simulink model "PID_DC_motor_control_linear"  (R2017a)
settings: Solver=ode45  StartTime=0.0  StopTime=50  RelTol=1e-5  EnableMultiTasking=on
libraries: simulink x1
settings Model: Creator=The MathWorks, Inc.  LastModifiedBy=hemma
settings DataIOCC: LimitDataPoints=on  SaveFormat=Array
settings OptimizationCC: ExpressionDepthLimit=2147483647  LifeSpan=inf
settings DebuggingCC: UnderspecifiedInitializationDetection=Classic  MergeDetectMultiDrivingBlocksExec=none  FcnCallInpInsideContextMsg=warning  AllowSymbolicDim=off  StateNameClashWarn=warning  SFUnexpectedBacktrackingDiag=warning  SFNoUnconditionalDefaultTransitionDiag=warning  SFExecutionAtInitializationDiag=none
settings HardwareCC: ProdBitPerPointer=32  ProdBitPerSizeT=32  ProdBitPerPtrDiffT=32  ProdLargestAtomicFloat=None  ProdIntDivRoundTo=Undefined  ProdEndianess=Unspecified  ProdWordSize=32  ProdHWDeviceType=32-bit Generic
settings ModelReferenceCC: PropagateSignalLabelsOutOfModel=off
settings GRTTargetCC: TargetLangStandard=C89/C90 (ANSI)  GeneratePreprocessorConditionals=Disable all  CombineOutputUpdateFcns=off  GRTInterface=on
settings ConfigComp: CovMetricSettings=dw  CovHtmlReporting=on  CovSaveCumulativeToWorkspaceVar=on  CovSaveSingleToWorkspaceVar=on  CovExternalEMLEnable=off  CovSFcnEnable=off

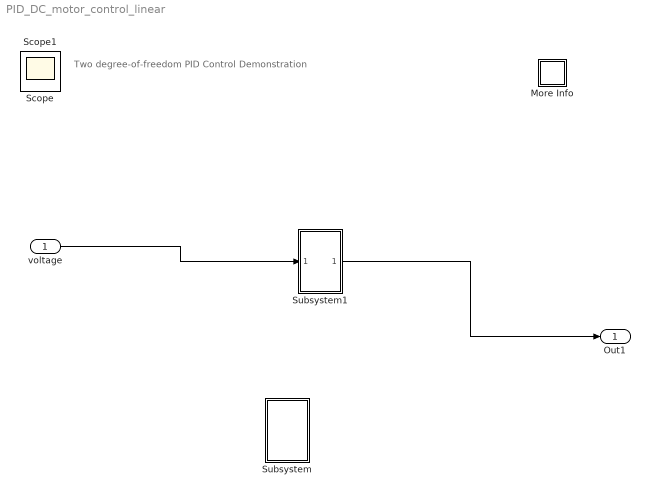
== system PID_DC_motor_control_linear ==
  note: Two degree-of-freedom PID Control Demonstration
  "voltage " : Inport
  More Info : Subsystem
      settings: OpenFcn=showdemo('sldemo_pid2dof')
      mask Display: disp('?')
  Subsystem : Subsystem
  Subsystem1 : Subsystem
  Out1 : Outport
  Scope : Scope
  Scope1 : Scope
  wires:
  "voltage "/1 -> Subsystem1/1("voltage ")
  Subsystem1/1(Out1) -> Out1/1

== system PID_DC_motor_control_linear/More Info ==

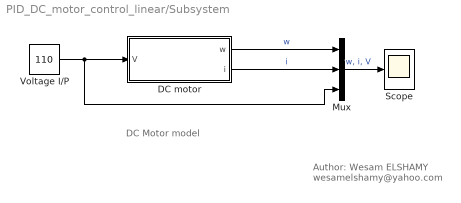
== system PID_DC_motor_control_linear/Subsystem ==
  note: Author: Wesam ELSHAMY
      | wesamelshamy@yahoo.com
  note: DC Motor model
  DC motor : Subsystem  mask(DC Motor){L=0.1, Kphi=0.3, J=0.1, b=0.01, R=2}
      mask help:
      | Takes the DC voltage as input, and outputs angular velocity (w) and current (i)
      | L => windings inductance		Kphi => emf constant
      | J => loads moment of inertial		b => viscous friction
      | R => windings resistance
      mask Display:
      | port_label('input', 1, 'V')
      | port_label('output', 2, 'i')
      | port_label('output', 1, 'w')
      | disp('DC Motor')
  Mux : Mux  Inputs=3
  Scope : Scope
  Voltage I/P : Constant  Value=110
  wires:
  DC motor/2(i) -> Mux/2  "i"
  Mux/1 -> Scope/1  "w, i, V"
  DC motor/1(w) -> Mux/1  "w"
  Voltage I/P/1 -> Mux/3, DC motor/1(V)

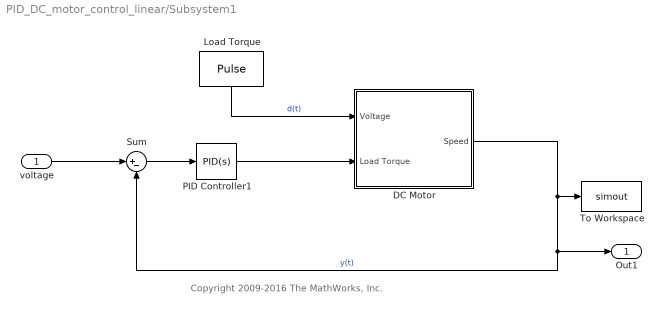
== system PID_DC_motor_control_linear/Subsystem1 ==
  note: Copyright 2009-2016 The MathWorks, Inc.
  "voltage " : Inport
  DC Motor : Subsystem  mask(DC Motor){R=2, L=0.5, Km=0.1, Kf=0.2, J=0.02, Kb=0.1}
      mask prompts: R "R (Ohms)"; L "L (Henrys)"; Km "Km (Torque Constant)"; Kf "Kf (Nms)"; J "J (kg.m^2/s^2)"; Kb "Kb (Back emf Constant)"
      mask help: An ideal model of a DC Motor
      mask Help: This is <b>more elaborate<b> help.
      mask Display: image(fullfile(matlabroot,'toolbox','simulink','simdemos','industrial','images','maskIconDCMotor.png'))
  Load Torque : DiscretePulseGenerator  PulseType=Time based  Amplitude=-20  Period=100  PulseWidth=50
  PID Controller1 : simulink/Continuous/PID Controller  Controller=PID  TimeDomain=Continuous-time  SampleTime=-1  IntegratorMethod=Forward Euler  FilterMethod=Forward Euler  Form=Parallel  UseFilter=on  ControllerParametersSource=internal  P=1.25  I=0  D=0.1  N=0  InitialConditionSource=internal  InitialConditionForIntegrator=0  InitialConditionForFilter=0  ExternalReset=none  LimitOutput=off  UpperSaturationLimit=inf  LowerSaturationLimit=-inf  LinearizeAsGain=on  AntiWindupMode=none  Kb=1  TrackingMode=off  Kt=1  PParamMin=[]  PParamMax=[]  IParamMin=[]  IParamMax=[]  DParamMin=[]  DParamMax=[]  NParamMin=[]  NParamMax=[]  KbParamMin=[]  KbParamMax=[]  KtParamMin=[]  KtParamMax=[]  POutMin=[]  POutMax=[]  IOutMin=[]  IOutMax=[]  DOutMin=[]  DOutMax=[]  NOutMin=[]  NOutMax=[]  KbOutMin=[]  KbOutMax=[]  KtOutMin=[]  KtOutMax=[]  IntegratorOutMin=[]  IntegratorOutMax=[]  FilterOutMin=[]  FilterOutMax=[]  SumOutMin=[]  SumOutMax=[]  SumI1OutMin=[]  SumI1OutMax=[]  SumI2OutMin=[]  SumI2OutMax=[]  SumI3OutMin=[]  SumI3OutMax=[]  SumDOutMin=[]  SumDOutMax=[]  SaturationOutMin=[]  SaturationOutMax=[]  IntegratorContinuousStateAttributes=''  IntegratorStateMustResolveToSignalObject=off  IntegratorRTWStateStorageClass=Auto  FilterContinuousStateAttributes=''  FilterStateMustResolveToSignalObject=off  FilterRTWStateStorageClass=Auto  DifferentiatorICPrevScaledInput=0  DifferentiatorOutMin=[]  DifferentiatorOutMax=[]  InitialConditionSetting=State (most efficient)
  Sum : Sum  Inputs=|+-
  To Workspace : ToWorkspace  VariableName=simout  SaveFormat=Structure With Time  SampleTime=-1
  Out1 : Outport
  wires:
  Load Torque/1 -> DC Motor/1(Voltage)  "d(t)"
  "voltage "/1 -> Sum/1
  PID Controller1/1 -> DC Motor/2(Load Torque)
  DC Motor/1(Speed) -> To Workspace/1, Out1/1, Sum/2  "y(t)"
  Sum/1 -> PID Controller1/1

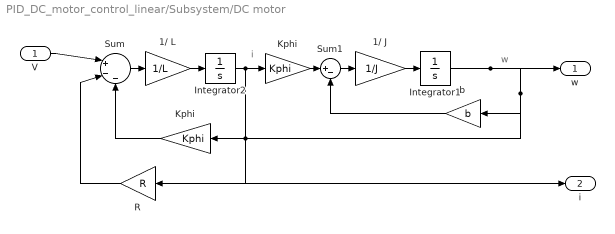
== system PID_DC_motor_control_linear/Subsystem/DC motor ==
  note: w
  note: i
  V : Inport
  1/ J : Gain  Gain=1/J
  1/ L : Gain  Gain=1/L
  Integrator1 : Integrator
  Integrator2 : Integrator
  Kphi : Gain  Gain=Kphi
  "Kphi " : Gain  Gain=Kphi
  R : Gain  Gain=R
  Sum : Sum  Inputs=|+--
  Sum1 : Sum  Inputs=|+-
  b : Gain  Gain=b
  w : Outport
  i : Outport  Port=2
  wires:
  R/1 -> Sum/2
  "Kphi "/1 -> Sum/3
  b/1 -> Sum1/2
  Integrator1/1 -> w/1, b/1, "Kphi "/1
  1/ J/1 -> Integrator1/1
  Sum1/1 -> 1/ J/1
  Kphi/1 -> Sum1/1
  Integrator2/1 -> i/1, R/1, Kphi/1
  1/ L/1 -> Integrator2/1
  Sum/1 -> 1/ L/1
  V/1 -> Sum/1

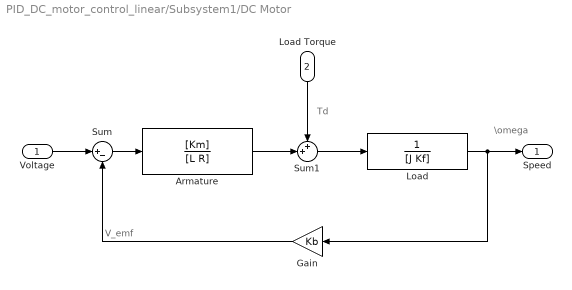
== system PID_DC_motor_control_linear/Subsystem1/DC Motor ==
  note: \omega
  note: V_emf
  note: Td
  Voltage : Inport
  Load Torque : Inport  Port=2
  Armature : TransferFcn  Numerator=[Km]  Denominator=[L R]
  Gain : Gain  Gain=Kb
  Load : TransferFcn  Denominator=[J Kf]
  Sum : Sum  Inputs=|+-
  Sum1 : Sum  Inputs=++|
  Speed : Outport
  wires:
  Load/1 -> Speed/1, Gain/1
  Load Torque/1 -> Sum1/1
  Armature/1 -> Sum1/2
  Sum1/1 -> Load/1
  Sum/1 -> Armature/1
  Voltage/1 -> Sum/1
  Gain/1 -> Sum/2
